simulink model "task4sim"  (R2022b)
settings: Solver=VariableStepAuto  StartTime=0.0  StopTime=90.0  RelTol=1e-3
values from neighbouring files (symbols this model uses):
  B_c = Bc_c    (= 900)    [task1.m]    (also in task4.m)
  B_s = 700    [task1.m]    (also in task4.m)
  B_sb = 300    [task1.m]    (also in task4.m)
  K_c = Kc_c    (= 8000)    [task1.m]    (also in task4.m)
  K_s = 2200    [task1.m]    (also in task4.m)
  K_t = 120000    [task1.m]    (also in task4.m)
  M_c = 250    [task1.m]    (also in task4.m)
  M_s = 100    [task1.m]    (also in task4.m)
  M_t = 50    [task1.m]    (also in task4.m)
settings Model: Creator=daddal  LastModifiedBy=daddal
settings HardwareCC: ProdBitPerLong=64  ProdHWDeviceType=Intel->x86-64 (Mac OS X)

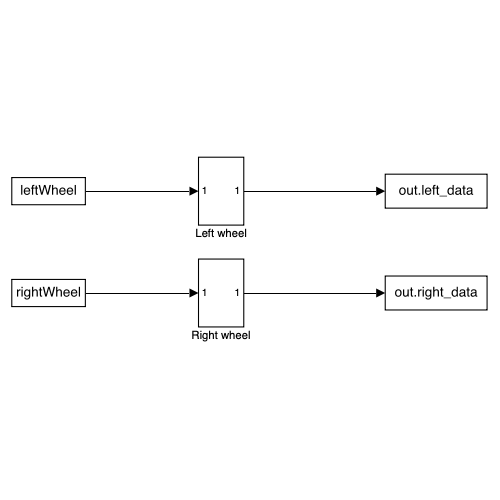
[thumbnail: Simulink's stored preview of the top-level diagram]
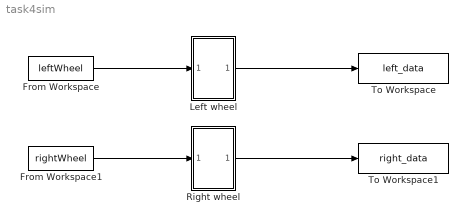
== system task4sim ==
  From Workspace : FromWorkspace  VariableName=leftWheel  OutputAfterFinalValue=Setting to zero
  From Workspace1 : FromWorkspace  VariableName=rightWheel  OutputAfterFinalValue=Setting to zero
  Left wheel : Subsystem
  Right wheel : Subsystem
  To Workspace : ToWorkspace  VariableName=left_data  SaveFormat=Timeseries  SampleTime=-1
  To Workspace1 : ToWorkspace  VariableName=right_data  SaveFormat=Timeseries  SampleTime=-1
  wires:
  From Workspace/1 -> Left wheel/1(In1)
  From Workspace1/1 -> Right wheel/1(In1)
  Right wheel/1(Out1) -> To Workspace1/1
  Left wheel/1(Out1) -> To Workspace/1

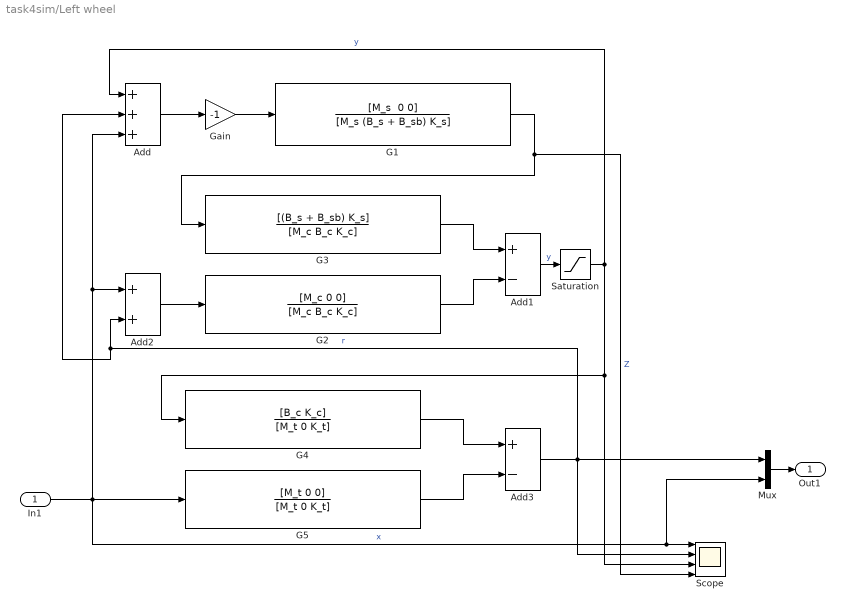
== system task4sim/Left wheel ==
  In1 : Inport
  Add : Sum  Inputs=+++
  Add1 : Sum  Inputs=+-
  Add2 : Sum
  Add3 : Sum  Inputs=+-
  G1 : TransferFcn  Numerator="[M_s  0 0]"  Denominator=[M_s (B_s + B_sb) K_s]  ParameterTunability=Unconstrained
  G2 : TransferFcn  Numerator=[M_c 0 0]  Denominator=[M_c B_c K_c]
  G3 : TransferFcn  Numerator=[(B_s + B_sb) K_s]  Denominator=[M_c B_c K_c]
  G4 : TransferFcn  Numerator=[B_c K_c]  Denominator=[M_t 0 K_t]
  G5 : TransferFcn  Numerator=[M_t 0 0]  Denominator=[M_t 0 K_t]
  Gain : Gain  Gain=-1
  Mux : Mux  Inputs=2
  Saturation : Saturate  UpperLimit=0.02  LowerLimit=-0.02
  Scope : Scope  NumInputPorts=4
  Out1 : Outport
  wires:
  Add/1 -> Gain/1
  G3/1 -> Add1/1
  G4/1 -> Add3/1
  G5/1 -> Add3/2
  G2/1 -> Add1/2
  Add1/1 -> Saturation/1  "y"
  Add2/1 -> G2/1
  Add3/1 -> Add/2, Add2/2, Mux/1, Scope/2  "r"
  Gain/1 -> G1/1
  In1/1 -> G5/1, Mux/2, Scope/1, Add/3, Add2/1  "x"
  G1/1 -> Scope/4, G3/1  "Z"
  Saturation/1 -> G4/1, Scope/3, Add/1  "y"
  Mux/1 -> Out1/1

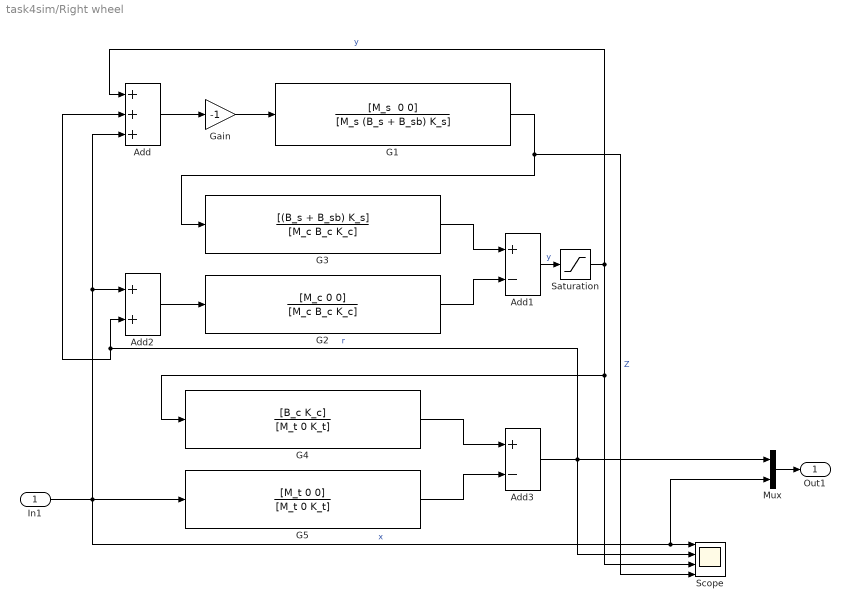
== system task4sim/Right wheel ==
  In1 : Inport
  Add : Sum  Inputs=+++
  Add1 : Sum  Inputs=+-
  Add2 : Sum
  Add3 : Sum  Inputs=+-
  G1 : TransferFcn  Numerator="[M_s  0 0]"  Denominator=[M_s (B_s + B_sb) K_s]  ParameterTunability=Unconstrained
  G2 : TransferFcn  Numerator=[M_c 0 0]  Denominator=[M_c B_c K_c]
  G3 : TransferFcn  Numerator=[(B_s + B_sb) K_s]  Denominator=[M_c B_c K_c]
  G4 : TransferFcn  Numerator=[B_c K_c]  Denominator=[M_t 0 K_t]
  G5 : TransferFcn  Numerator=[M_t 0 0]  Denominator=[M_t 0 K_t]
  Gain : Gain  Gain=-1
  Mux : Mux  Inputs=2
  Saturation : Saturate  UpperLimit=0.02  LowerLimit=-0.02
  Scope : Scope  NumInputPorts=4
  Out1 : Outport
  wires:
  Add/1 -> Gain/1
  G3/1 -> Add1/1
  G4/1 -> Add3/1
  G5/1 -> Add3/2
  G2/1 -> Add1/2
  Add1/1 -> Saturation/1  "y"
  Add2/1 -> G2/1
  Gain/1 -> G1/1
  G1/1 -> Scope/4, G3/1  "Z"
  Saturation/1 -> G4/1, Scope/3, Add/1  "y"
  Mux/1 -> Out1/1
  In1/1 -> G5/1, Mux/2, Scope/1, Add/3, Add2/1  "x"
  Add3/1 -> Mux/1, Scope/2, Add/2, Add2/2  "r"
